simulink model "LANDER_HOT"  (R2021a)
settings: Solver=VariableStepAuto  StartTime=0.0  StopTime=43200  RelTol=1e-3
libraries: fl_lib x22, nesl_utility x4
settings Model: Creator=dinen  LastModifiedBy=dinen

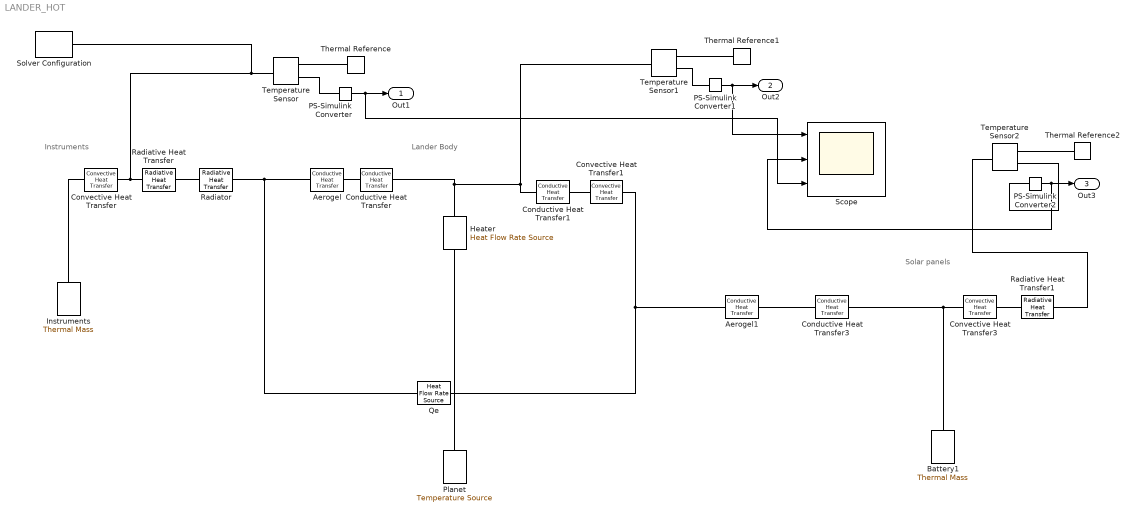
== system LANDER_HOT ==
  note: Solar panels
  note: Lander Body
  note: Instruments
  Aerogel : fl_lib/Thermal/Thermal Elements/Conductive Heat Transfer  area=4.305 m^2  thickness=0.016 m  th_cond=0.015 W/(m*K)  T_specify=off  T_priority=None  T=0 K  T_nominal_specify=off  T_nominal_unit=K  T_nominal_value=1  Q_specify=off  Q_priority=None  Q=0 W  Q_nominal_specify=off  Q_nominal_unit=W  Q_nominal_value=1
  Aerogel1 : fl_lib/Thermal/Thermal Elements/Conductive Heat Transfer  area=0.05 m^2  thickness=0.016 m  th_cond=0.015 W/(m*K)  T_specify=off  T_priority=None  T=0 K  T_nominal_specify=off  T_nominal_unit=K  T_nominal_value=1  Q_specify=off  Q_priority=None  Q=0 W  Q_nominal_specify=off  Q_nominal_unit=W  Q_nominal_value=1
  Battery1 : fl_lib/Thermal/Thermal Elements/Thermal Mass  mass=10 kg  sp_heat=460 J/kg/K  T_specify=off  T_priority=None  T=273 K  T_nominal_specify=off  T_nominal_unit=K  T_nominal_value=1  Q_specify=off  Q_priority=None  Q=167.4 W  Q_nominal_specify=off  Q_nominal_unit=W  Q_nominal_value=1
  Conductive Heat Transfer : fl_lib/Thermal/Thermal Elements/Conductive Heat Transfer  area=1.015 m^2  thickness=0.063 m  th_cond=130 W/(m*K)  T_specify=off  T_priority=None  T=0 K  T_nominal_specify=off  T_nominal_unit=K  T_nominal_value=1  Q_specify=off  Q_priority=None  Q=0 W  Q_nominal_specify=off  Q_nominal_unit=W  Q_nominal_value=1
  Conductive Heat Transfer1 : fl_lib/Thermal/Thermal Elements/Conductive Heat Transfer  area=4.305 m^2  thickness=0.063 m  th_cond=130 W/(m*K)  T_specify=off  T_priority=None  T=0 K  T_nominal_specify=off  T_nominal_unit=K  T_nominal_value=1  Q_specify=off  Q_priority=None  Q=0 W  Q_nominal_specify=off  Q_nominal_unit=W  Q_nominal_value=1
  Conductive Heat Transfer3 : fl_lib/Thermal/Thermal Elements/Conductive Heat Transfer  area=0.05 m^2  thickness=0.1 m  th_cond=120 W/(m*K)  T_specify=off  T_priority=None  T=0 K  T_nominal_specify=off  T_nominal_unit=K  T_nominal_value=1  Q_specify=off  Q_priority=None  Q=0 W  Q_nominal_specify=off  Q_nominal_unit=W  Q_nominal_value=1
  Convective Heat Transfer : fl_lib/Thermal/Thermal Elements/Convective Heat Transfer  area=1.015 m^2  heat_tr_coeff=4 W/(m^2 * K)  T_specify=off  T_priority=None  T=0 K  T_nominal_specify=off  T_nominal_unit=K  T_nominal_value=1  Q_specify=off  Q_priority=None  Q=0 W  Q_nominal_specify=off  Q_nominal_unit=W  Q_nominal_value=1
  Convective Heat Transfer1 : fl_lib/Thermal/Thermal Elements/Convective Heat Transfer  area=4.305 m^2  heat_tr_coeff=4 W/(m^2 * K)  T_specify=off  T_priority=None  T=0 K  T_nominal_specify=off  T_nominal_unit=K  T_nominal_value=1  Q_specify=off  Q_priority=None  Q=0 W  Q_nominal_specify=off  Q_nominal_unit=W  Q_nominal_value=1
  Convective Heat Transfer3 : fl_lib/Thermal/Thermal Elements/Convective Heat Transfer  area=14.2 m^2  heat_tr_coeff=4 W/(m^2 * K)  T_specify=off  T_priority=None  T=0 K  T_nominal_specify=off  T_nominal_unit=K  T_nominal_value=1  Q_specify=off  Q_priority=None  Q=0 W  Q_nominal_specify=off  Q_nominal_unit=W  Q_nominal_value=1
  Heater : fl_lib/Thermal/Thermal Sources/Heat Flow Rate Source  heat_flow=0 W
      settings: SourceProductBaseCode=SS  InternalSimscapePortConfiguration="{\"Bottom\":[],\"Left\":[{\"id\":\"B\",\"label\":\"B\",\"type\":\"foundation.thermal.thermal\"}],\"Right\":[{\"id\":\"A\",\"label\":\"A\",\"type\":\"foundation.thermal.thermal\"}],\"Top\":[]}"
  Instruments : fl_lib/Thermal/Thermal Elements/Thermal Mass  mass=26.3 kg  sp_heat=903 J/kg/K  T_specify=on  T_priority=High  T=273 K  T_nominal_specify=off  T_nominal_unit=K  T_nominal_value=1  Q_specify=off  Q_priority=None  Q=0 W  Q_nominal_specify=off  Q_nominal_unit=W  Q_nominal_value=1
  PS-Simulink Converter : nesl_utility/PS-Simulink Converter  PhysicalDomain=network_engine_domain  SubClassName=ps_output  LeftPortType=input  RightPortType=output  PseudoPeriodic=off  Frequencies=[]  Unit=inherit  AffineConversion=off
      settings: SourceProductBaseCode=PW,SS
  PS-Simulink Converter1 : nesl_utility/PS-Simulink Converter  PhysicalDomain=network_engine_domain  SubClassName=ps_output  LeftPortType=input  RightPortType=output  PseudoPeriodic=off  Frequencies=[]  Unit=inherit  AffineConversion=off
      settings: SourceProductBaseCode=PW,SS
  PS-Simulink Converter2 : nesl_utility/PS-Simulink Converter  PhysicalDomain=network_engine_domain  SubClassName=ps_output  LeftPortType=input  RightPortType=output  PseudoPeriodic=off  Frequencies=[]  Unit=inherit  AffineConversion=off
      settings: SourceProductBaseCode=PW,SS
  Planet : fl_lib/Thermal/Thermal Sources/Temperature Source  temperature=303 K
  Qe : fl_lib/Thermal/Thermal Sources/Heat Flow Rate Source  heat_flow=127.1 W
      settings: SourceProductBaseCode=SS  InternalSimscapePortConfiguration="{\"Bottom\":[],\"Left\":[{\"id\":\"B\",\"label\":\"B\",\"type\":\"foundation.thermal.thermal\"}],\"Right\":[{\"id\":\"A\",\"label\":\"A\",\"type\":\"foundation.thermal.thermal\"}],\"Top\":[]}"
  Radiative Heat Transfer : fl_lib/Thermal/Thermal Elements/Radiative Heat Transfer  area=1.015 m^2  rad_tr_coeff=0.5684 W/(m^2*K^4)  T_specify=off  T_priority=None  T=0 K  T_nominal_specify=off  T_nominal_unit=K  T_nominal_value=1  Q_specify=off  Q_priority=None  Q=0 W  Q_nominal_specify=off  Q_nominal_unit=W  Q_nominal_value=1
      settings: SourceProductBaseCode=SS  InternalSimscapePortConfiguration="{\"Bottom\":[],\"Left\":[{\"id\":\"A\",\"label\":\"A\",\"type\":\"foundation.thermal.thermal\"}],\"Right\":[{\"id\":\"B\",\"label\":\"B\",\"type\":\"foundation.thermal.thermal\"}],\"Top\":[]}"
  Radiative Heat Transfer1 : fl_lib/Thermal/Thermal Elements/Radiative Heat Transfer  area=14.2 m^2  rad_tr_coeff=6.958 W/(m^2*K^4)  T_specify=off  T_priority=None  T=0 K  T_nominal_specify=off  T_nominal_unit=K  T_nominal_value=1  Q_specify=off  Q_priority=None  Q=0 W  Q_nominal_specify=off  Q_nominal_unit=W  Q_nominal_value=1
      settings: SourceProductBaseCode=SS  InternalSimscapePortConfiguration="{\"Bottom\":[],\"Left\":[{\"id\":\"A\",\"label\":\"A\",\"type\":\"foundation.thermal.thermal\"}],\"Right\":[{\"id\":\"B\",\"label\":\"B\",\"type\":\"foundation.thermal.thermal\"}],\"Top\":[]}"
  Radiator : fl_lib/Thermal/Thermal Elements/Radiative Heat Transfer  area=0.45 m^2  rad_tr_coeff=0.252 W/(m^2*K^4)  T_specify=off  T_priority=None  T=0 K  T_nominal_specify=off  T_nominal_unit=K  T_nominal_value=1  Q_specify=off  Q_priority=None  Q=0 W  Q_nominal_specify=off  Q_nominal_unit=W  Q_nominal_value=1
      settings: SourceProductBaseCode=SS  InternalSimscapePortConfiguration="{\"Bottom\":[],\"Left\":[{\"id\":\"A\",\"label\":\"A\",\"type\":\"foundation.thermal.thermal\"}],\"Right\":[{\"id\":\"B\",\"label\":\"B\",\"type\":\"foundation.thermal.thermal\"}],\"Top\":[]}"
  Scope : Scope  NumInputPorts=3
  Solver Configuration : nesl_utility/Solver Configuration  PhysicalDomain=network_engine_domain  SubClassName=solver  LeftPortType=input  RightPortType=generic  Tones=[]  Harmonics=[]  SimulateNoise=off  Profile=off  UseLocalSampling=off  EnableSwitchedLinearOptims=on  FrequencyDomain=off  UseCCode=off  RelTol=0.001  AbsTol=1e-06  MinStep=1e-09  ToWorkspace=off  RevertToSquareIcSolve=off  NumHomotopyIterations=100  PhasorMode=off  PhasorModeNumHarmonics=1  DoDC=off  ResidualTolerance=1e-09  UseLocalSolver=off  LocalSolverChoice=NE_BACKWARD_EULER_ADVANCER  LocalSolverSampleTime=0.001  DoFixedCost=off  MaxNonlinIter=3  MaxModeIter=2  ComputeImpulses=off  ImpulseIterations=2  LinearAlgebra=auto  EquationFormulation=NE_TIME_EF  DelaysMemoryBudget=1024  AutomaticFiltering=on  FilteringTimeConstant=0.001  PartitionStorageMethod=AS_NEEDED  PartitionMemoryBudget=1024  PartitionMethod=ROBUST
      settings: SourceProductBaseCode=PW,SS
  Temperature Sensor : fl_lib/Thermal/Thermal Sensors/Temperature Sensor
  Temperature Sensor1 : fl_lib/Thermal/Thermal Sensors/Temperature Sensor
  Temperature Sensor2 : fl_lib/Thermal/Thermal Sensors/Temperature Sensor
  Thermal Reference : fl_lib/Thermal/Thermal Elements/Thermal Reference
  Thermal Reference1 : fl_lib/Thermal/Thermal Elements/Thermal Reference
  Thermal Reference2 : fl_lib/Thermal/Thermal Elements/Thermal Reference
  Out1 : Outport
  Out2 : Outport  Port=2
  Out3 : Outport  Port=3
  wires:
  PS-Simulink Converter1/1 -> Scope/1, Out2/1
  PS-Simulink Converter/1 -> Scope/3, Out1/1
  PS-Simulink Converter2/1 -> Scope/2, Out3/1
  connections:
  Convective Heat Transfer/RConn1 -- Solver Configuration/RConn1 -- Temperature Sensor/LConn1 -- Radiative Heat Transfer/LConn1
  Qe/RConn1 -- Aerogel/LConn1 -- Radiator/RConn1
  Aerogel/RConn1 -- Conductive Heat Transfer/LConn1
  Heater/RConn1 -- Planet/LConn1
  Conductive Heat Transfer1/RConn1 -- Convective Heat Transfer1/LConn1
  Qe/LConn1 -- Aerogel1/LConn1 -- Convective Heat Transfer1/RConn1
  Temperature Sensor/RConn1 -- Thermal Reference/LConn1
  Temperature Sensor1/RConn1 -- Thermal Reference1/LConn1
  Temperature Sensor/RConn2 -- PS-Simulink Converter/LConn1
  Temperature Sensor1/RConn2 -- PS-Simulink Converter1/LConn1
  Convective Heat Transfer/LConn1 -- Instruments/LConn1
  Radiator/LConn1 -- Radiative Heat Transfer/RConn1
  Temperature Sensor1/LConn1 -- Conductive Heat Transfer/RConn1 -- Heater/LConn1 -- Conductive Heat Transfer1/LConn1
  Radiative Heat Transfer1/LConn1 -- Convective Heat Transfer3/RConn1
  Temperature Sensor2/RConn2 -- PS-Simulink Converter2/LConn1
  Temperature Sensor2/RConn1 -- Thermal Reference2/LConn1
  Temperature Sensor2/LConn1 -- Radiative Heat Transfer1/RConn1
  Battery1/LConn1 -- Convective Heat Transfer3/LConn1 -- Conductive Heat Transfer3/RConn1
  Aerogel1/RConn1 -- Conductive Heat Transfer3/LConn1
